simulink model "SINE_WAVE_ADD"  (R2020b)
settings: Solver=VariableStepAuto  StartTime=0.0  StopTime=10.0  RelTol=1e-3
settings Model: Creator=Raihan mahmud  LastModifiedBy=Raihan mahmud

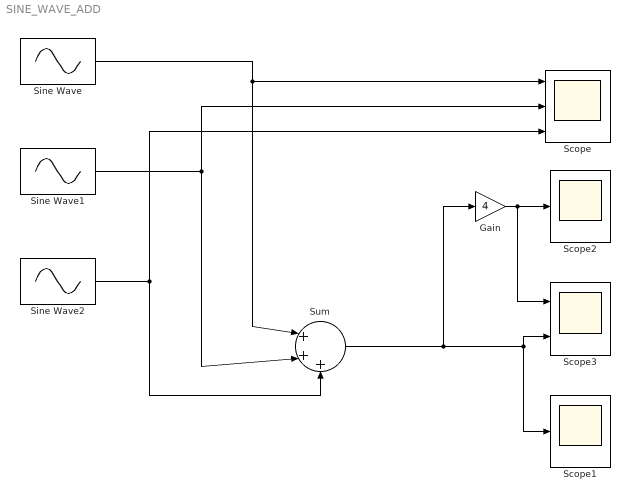
== system SINE_WAVE_ADD ==
  Gain : Gain  Gain=4
  Scope : Scope  NumInputPorts=3
  Scope1 : Scope
  Scope2 : Scope
  Scope3 : Scope  NumInputPorts=2
  Sine Wave : Sin  SampleTime=0
  Sine Wave1 : Sin  Amplitude=2  Frequency=2  SampleTime=0
  Sine Wave2 : Sin  Amplitude=3  Frequency=3  SampleTime=0
  Sum : Sum  Inputs=|+++
  wires:
  Sine Wave/1 -> Sum/1, Scope/1
  Sine Wave1/1 -> Sum/2, Scope/2
  Sine Wave2/1 -> Sum/3, Scope/3
  Gain/1 -> Scope3/1, Scope2/1
  Sum/1 -> Gain/1, Scope3/2, Scope1/1
